simulink model "untitled"  (R2019b)
settings: Solver=VariableStepAuto  StartTime=0.0  StopTime=2  RelTol=1e-3
undefined symbols (not defined in the file): Ion, Lithium, sigbuilder_block
libraries: powerlib x38, simulink x10, electricdrivelib x4, re_lib x2, mpclib x1
settings Model: Creator=ADHI  LastModifiedBy=ADHI
settings SolverCC: AlgebraicLoopSolver=LineSearch

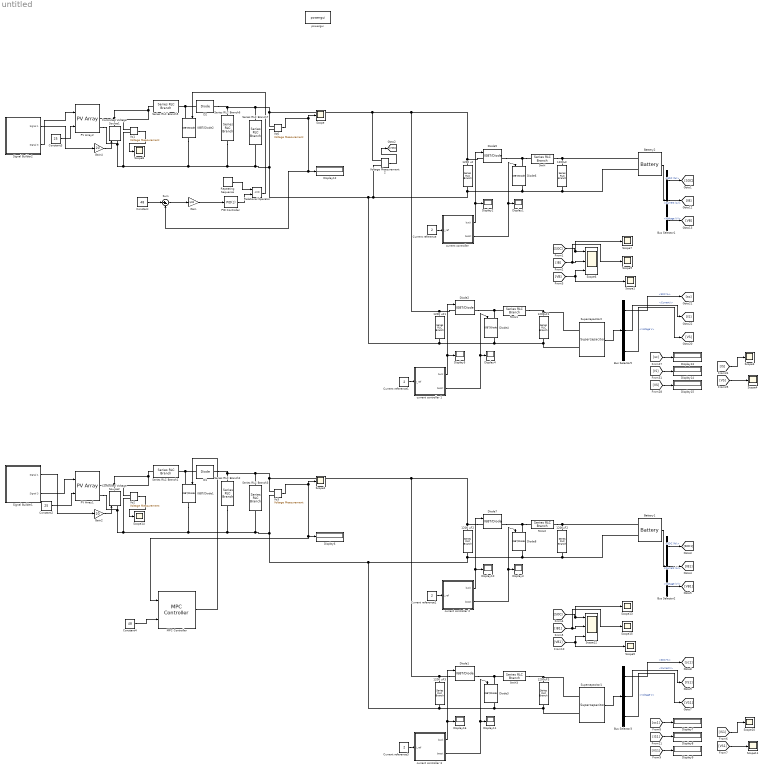
== system untitled ==
  1200 uF : powerlib/Elements/Series RLC Branch  LConnTagsString=__new0  RConnTagsString=__new0  BranchType=RC  Resistance=0.1  Inductance=3e-3  SetiL0=off  InitialCurrent=0  Capacitance=1200e-6  Setx0=off  InitialVoltage=0  Measurements=None
  1200 uF1 : powerlib/Elements/Series RLC Branch  LConnTagsString=__new0  RConnTagsString=__new0  BranchType=RC  Resistance=1  Inductance=3e-3  SetiL0=off  InitialCurrent=0  Capacitance=120e-6  Setx0=off  InitialVoltage=0  Measurements=None
  1200 uF2 : powerlib/Elements/Series RLC Branch  LConnTagsString=__new0  RConnTagsString=__new0  BranchType=RC  Resistance=0.1  Inductance=3e-3  SetiL0=off  InitialCurrent=0  Capacitance=1200e-6  Setx0=off  InitialVoltage=0  Measurements=None
  1200 uF3 : powerlib/Elements/Series RLC Branch  LConnTagsString=__new0  RConnTagsString=__new0  BranchType=RC  Resistance=1  Inductance=3e-3  SetiL0=off  InitialCurrent=0  Capacitance=120e-6  Setx0=off  InitialVoltage=0  Measurements=None
  1200uF : powerlib/Elements/Series RLC Branch  LConnTagsString=__new0  RConnTagsString=__new0  BranchType=C  Resistance=1  Inductance=3e-3  SetiL0=off  InitialCurrent=0  Capacitance=1200e-6  Setx0=off  InitialVoltage=0  Measurements=None
  1200uF1 : powerlib/Elements/Series RLC Branch  LConnTagsString=__new0  RConnTagsString=__new0  BranchType=C  Resistance=1  Inductance=3e-3  SetiL0=off  InitialCurrent=0  Capacitance=120e-6  Setx0=off  InitialVoltage=0  Measurements=None
  1200uF2 : powerlib/Elements/Series RLC Branch  LConnTagsString=__new0  RConnTagsString=__new0  BranchType=C  Resistance=1  Inductance=3e-3  SetiL0=off  InitialCurrent=0  Capacitance=1200e-6  Setx0=off  InitialVoltage=0  Measurements=None
  1200uF3 : powerlib/Elements/Series RLC Branch  LConnTagsString=__new0  RConnTagsString=__new0  BranchType=C  Resistance=1  Inductance=3e-3  SetiL0=off  InitialCurrent=0  Capacitance=120e-6  Setx0=off  InitialVoltage=0  Measurements=None
  9mH : powerlib/Elements/Series RLC Branch  LConnTagsString=__new0  RConnTagsString=__new0  BranchType=L  Resistance=1  Inductance=9e-3  SetiL0=off  InitialCurrent=0  Capacitance=1e-6  Setx0=off  InitialVoltage=0  Measurements=None
  9mH1 : powerlib/Elements/Series RLC Branch  LConnTagsString=__new0  RConnTagsString=__new0  BranchType=L  Resistance=1  Inductance=9e-6  SetiL0=off  InitialCurrent=0  Capacitance=1e-6  Setx0=off  InitialVoltage=0  Measurements=None
  9mH2 : powerlib/Elements/Series RLC Branch  LConnTagsString=__new0  RConnTagsString=__new0  BranchType=L  Resistance=1  Inductance=9e-3  SetiL0=off  InitialCurrent=0  Capacitance=1e-6  Setx0=off  InitialVoltage=0  Measurements=None
  9mH3 : powerlib/Elements/Series RLC Branch  LConnTagsString=__new0  RConnTagsString=__new0  BranchType=L  Resistance=1  Inductance=9e-6  SetiL0=off  InitialCurrent=0  Capacitance=1e-6  Setx0=off  InitialVoltage=0  Measurements=None
  Battery1 : electricdrivelib/Extra Sources/Battery  BatType=Lithium-Ion  ShowTempParam=off  ThermalPreset=no  ShowAgeParam=off  NomV=1.2  NomQ=6.5  SOC=50  Batt_Tr=1e-6  PresetModel=off  MaxQ=7  MinV=50  FullV=1.39  Dis_rate=1.3  R=2  Normal_OP=6.25  expZone=[1.28,1.3]  current=[1.5 3 6]  Units=Time  Tci=20  NomT=20  T2=-30  MaxQ2=4.8  FullV2=7.1  Normal_OP2=5.655  expZone2="[6.58           1]"  Rca=0.6  ti=2000  Dp=0  Neq0=0  Tsim=1e6  Ta1=25  Qeol=5.4*0.9  Reol=0.013333*1.2  Char_age=[2.3478, 3]  Dis_age=[2.3478, 10]  N1=1500  N2=10500  N3=1000  N4=1400  Ta2=45  N5=950
      settings: SourceProductName=Simscape Electrical
  Battery2 : electricdrivelib/Extra Sources/Battery  BatType=Lithium-Ion  ShowTempParam=off  ThermalPreset=no  ShowAgeParam=off  NomV=1.2  NomQ=6.5  SOC=50  Batt_Tr=1e-6  PresetModel=off  MaxQ=7  MinV=50  FullV=1.39  Dis_rate=1.3  R=2  Normal_OP=6.25  expZone=[1.28,1.3]  current=[1.5 3 6]  Units=Time  Tci=20  NomT=20  T2=-30  MaxQ2=4.8  FullV2=7.1  Normal_OP2=5.655  expZone2="[6.58           1]"  Rca=0.6  ti=2000  Dp=0  Neq0=0  Tsim=1e6  Ta1=25  Qeol=5.4*0.9  Reol=0.013333*1.2  Char_age=[2.3478, 3]  Dis_age=[2.3478, 10]  N1=1500  N2=10500  N3=1000  N4=1400  Ta2=45  N5=950
      settings: SourceProductName=Simscape Electrical
  Bus Selector1 : BusSelector  OutputSignals=SOC (%),Current (A),Voltage (V)
  Bus Selector2 : BusSelector  OutputSignals=SOC (%),Current (A),Voltage (V)
  Bus Selector3 : BusSelector  OutputSignals=SOC %,Current I,Voltage V
  Bus Selector5 : BusSelector  OutputSignals=SOC %,Current I,Voltage V
  Constant : Constant  Value=48
  Constant2 : Constant  Value=25
  Constant3 : Constant  Value=25
  Constant4 : Constant  Value=48
  Controlled Voltage Source1 : powerlib/Electrical Sources/Controlled Voltage Source  Initialize=on  Source_Type=DC  Amplitude=5  Phase=0  Frequency=0  Measurements=None
      settings: SourceProductName=Simscape Electrical
  Controlled Voltage Source2 : powerlib/Electrical Sources/Controlled Voltage Source  Initialize=on  Source_Type=DC  Amplitude=5  Phase=0  Frequency=0  Measurements=None
      settings: SourceProductName=Simscape Electrical
  Current reference{,1..3} (4 alike) : Constant  Value=2
  D1 : powerlib/Power Electronics/Diode  Ron=0.001  Lon=0  Vf=0.001  IC=0  UseSnubber=off  Rs=500  Cs=250e-9  Measurements=off
      settings: SourceProductName=Simscape Electrical
  D2 : powerlib/Power Electronics/Diode  Ron=0.001  Lon=0  Vf=0.001  IC=0  UseSnubber=off  Rs=500  Cs=250e-9  Measurements=off
      settings: SourceProductName=Simscape Electrical
  Diode{1..8} (8 alike) : powerlib/Power Electronics/IGBT//Diode  Ron=1e-3  Rs=1e5  Cs=inf  Measurements=on
  Display{1..16} (16 alike) : Display
  Gain : Gain  Gain=1/20
  Gain2 : Gain  Gain=20
  Gain4 : Gain  Gain=20
  IGBT/Diode1 : powerlib/Power Electronics/IGBT//Diode  Ron=1e-3  Rs=1e5  Cs=inf  Measurements=off
      settings: SourceProductName=Simscape Electrical
  IGBT/Diode2 : powerlib/Power Electronics/IGBT//Diode  Ron=1e-3  Rs=1e5  Cs=inf  Measurements=off
      settings: SourceProductName=Simscape Electrical
  MPC Controller : mpclib/MPC Controller  SCDEnableBlockLinearizationSpecification=on  is_multiple=0  enable_value=0  return_u0=off  updateMPCinCallerWorkspace=on  md_inport=off  mv_inport=off  uref_inport=off  return_cost=off  return_mvseq=off  return_qpstatus=off  return_xseq=off  return_state=off  return_ovseq=off  state_inport=off  umin_inport=off  umax_inport=off  ymin_inport=off  ymax_inport=off  cc_inport=off  ywt_inport=off  uwt_inport=off  duwt_inport=off  rhoeps_inport=off  pm_inport=off  MaximumP=10  HorizonChoice=FixedHorizon  n_ts=1  n_p=10  n_mv=1  n_md=1  n_ud=0  n_mo=1  n_uo=0  BlockDataType=double  SampleTimeInherited=off  switch_inport=off
  PID Controller : simulink/Continuous/PID Controller  Controller=PID  Form=Parallel  TimeDomain=Discrete-time  SampleTime=-1  IntegratorMethod=Forward Euler  FilterMethod=Forward Euler  ControllerParametersSource=internal  P=0.7  I=100  D=0  UseFilter=on  N=100  TunerSelectOption=Transfer Function Based (PID Tuner App)  InitialConditionSource=internal  InitialConditionForIntegrator=0  InitialConditionForFilter=0  DifferentiatorICPrevScaledInput=0  ExternalReset=none  TrackingMode=off  Kt=1  LimitOutput=on  UpperSaturationLimit=0.9  LowerSaturationLimit=0.1  LinearizeAsGain=on  AntiWindupMode=none  Kb=1  POutMin=[]  POutMax=[]  IOutMin=[]  IOutMax=[]  DOutMin=[]  DOutMax=[]  NOutMin=[]  NOutMax=[]  SumOutMin=[]  SumOutMax=[]  SaturationOutMin=[]  SaturationOutMax=[]  PParamMin=[]  PParamMax=[]  IParamMin=[]  IParamMax=[]  DParamMin=[]  DParamMax=[]  NParamMin=[]  NParamMax=[]  KbParamMin=[]  KbParamMax=[]  KtParamMin=[]  KtParamMax=[]  KbOutMin=[]  KbOutMax=[]  KtOutMin=[]  KtOutMax=[]  IntegratorOutMin=[]  IntegratorOutMax=[]  FilterOutMin=[]  FilterOutMax=[]  SumI1OutMin=[]  SumI1OutMax=[]  SumI2OutMin=[]  SumI2OutMax=[]  SumI3OutMin=[]  SumI3OutMax=[]  SumI4OutMin=[]  SumI4OutMax=[]  SumDOutMin=[]  SumDOutMax=[]  DifferentiatorOutMin=[]  DifferentiatorOutMax=[]  FilterDiffOutCoefMin=[]  FilterDiffOutCoefMax=[]  ReciprocalOutMin=[]  ReciprocalOutMax=[]  SumDenOutMin=[]  SumDenOutMax=[]  SumNumOutMin=[]  SumNumOutMax=[]  DivideOutMin=[]  DivideOutMax=[]  IntegratorContinuousStateAttributes=''  IntegratorStateMustResolveToSignalObject=off  IntegratorRTWStateStorageClass=Auto  FilterContinuousStateAttributes=''  FilterStateMustResolveToSignalObject=off  FilterRTWStateStorageClass=Auto  ParallelPVariant=InternalParameters  IdealPVariant=Disabled  IVariant=InternalParameters  DVariant=InternalParameters  IntegratorVariant=Discrete  SatVariant=Enabled  AWVariant=Passthrough  PCopyVariant=Disabled  TRVariant=Disabled  FdbkBlocksVariant=Forward  IdealPFdbkVariant=Disabled  SatFdbkVariant=Disabled  DerivativeFilterVariant=ForwardEulerFilter  NVariant=InternalParameters  NCopyVariant=Disabled  FilterICVariant=InternalICsFilter  IntegratorICVariant=InternalICs  ExternalResetVariant=Disabled  TRSumVariant=Passthrough  SumFdbkVariant=Disabled  SumVariant=Sum_PID
  PV Array1 : re_lib/Solar/PV Array  Npar=1  Nser=2  PlotType=array @ 1000 W/m2 & specified temperatures  S_vec="[ 1000  500  100 ]"  Temp_C_vec="[ 45 25  ]"  ModuleName=1Soltech 1STH-340-WH  PlotWhenSelected=off  Pm=339.78  Ncell=80  Voc=51.1  Isc=9.12  Vm=42  Im=8.09  beta_Voc_pc=-0.36  alpha_Isc_pc=0.09  beta_Voc=-0.18396  alpha_Isc=0.008208  IL=9.1647  I0=3.1652e-10  nI=1.0358  Rsh=66.7455  Rs=0.32744  BAL=off  Tc=1e-6  Tfilter=5e-5
      settings: SourceProductName=Simscape Electrical
  PV Array2 : re_lib/Solar/PV Array  Npar=1  Nser=2  PlotType=array @ 1000 W/m2 & specified temperatures  S_vec="[ 1000  500  100 ]"  Temp_C_vec="[ 45 25  ]"  ModuleName=1Soltech 1STH-340-WH  PlotWhenSelected=off  Pm=339.78  Ncell=80  Voc=51.1  Isc=9.12  Vm=42  Im=8.09  beta_Voc_pc=-0.36  alpha_Isc_pc=0.09  beta_Voc=-0.18396  alpha_Isc=0.008208  IL=9.1647  I0=3.1652e-10  nI=1.0358  Rsh=66.7455  Rs=0.32744  BAL=off  Tc=1e-6  Tfilter=5e-5
      settings: SourceProductName=Simscape Electrical
  Relational Operator : RelationalOperator  Operator=<=  OutDataTypeStr=boolean  RndMeth=Simplest
  Repeating Sequence : simulink/Sources/Repeating Sequence  rep_seq_t=[0 0.00004]  rep_seq_y=[0 1]
  Scope{,1..5,7..11,13..15} (14 alike) : Scope
  Scope12 : Scope  NumInputPorts=3
  Scope6 : Scope  NumInputPorts=3
  Series RLC Branch1 : powerlib/Elements/Series RLC Branch  LConnTagsString=__new0  RConnTagsString=__new0  BranchType=L  Resistance=1  Inductance=150e-9  SetiL0=off  InitialCurrent=0  Capacitance=1e-6  Setx0=off  InitialVoltage=0  Measurements=None
      settings: SourceProductName=Simscape Electrical
  Series RLC Branch2 : powerlib/Elements/Series RLC Branch  LConnTagsString=__new0  RConnTagsString=__new0  BranchType=C  Resistance=1  Inductance=1e-3  SetiL0=off  InitialCurrent=0  Capacitance=360e-6  Setx0=off  InitialVoltage=0  Measurements=None
      settings: SourceProductName=Simscape Electrical
  Series RLC Branch3 : powerlib/Elements/Series RLC Branch  LConnTagsString=__new0  RConnTagsString=__new0  BranchType=R  Resistance=10  Inductance=1e-3  SetiL0=off  InitialCurrent=0  Capacitance=220e-6  Setx0=off  InitialVoltage=0  Measurements=None
      settings: SourceProductName=Simscape Electrical
  Series RLC Branch5 : powerlib/Elements/Series RLC Branch  LConnTagsString=__new0  RConnTagsString=__new0  BranchType=L  Resistance=1  Inductance=150e-9  SetiL0=off  InitialCurrent=0  Capacitance=1e-6  Setx0=off  InitialVoltage=0  Measurements=None
      settings: SourceProductName=Simscape Electrical
  Series RLC Branch6 : powerlib/Elements/Series RLC Branch  LConnTagsString=__new0  RConnTagsString=__new0  BranchType=C  Resistance=1  Inductance=1e-3  SetiL0=off  InitialCurrent=0  Capacitance=360e-6  Setx0=off  InitialVoltage=0  Measurements=None
      settings: SourceProductName=Simscape Electrical
  Series RLC Branch7 : powerlib/Elements/Series RLC Branch  LConnTagsString=__new0  RConnTagsString=__new0  BranchType=R  Resistance=10  Inductance=1e-3  SetiL0=off  InitialCurrent=0  Capacitance=220e-6  Setx0=off  InitialVoltage=0  Measurements=None
      settings: SourceProductName=Simscape Electrical
  Signal Builder1 : Subsystem  Tag=STV Subsys  LoadFcn=sigbuilder_block('load');  StartFcn=sigbuilder_block('start');  StopFcn=sigbuilder_block('stop');  ClipboardFcn=sigbuilder_block('clipboard');  mask(Sigbuilder block){tuvar=[0:10]}
      mask help: Simulink:masks:SigbuilderBlock_MD
      mask init:
      | if ~strcmp(get_param(bdroot(gcbh),'SimulationStatus'),'stopped') tuvar = sigbuilder_block('maskInit'); end
      settings: CopyFcn=sigbuilder_block('copy');  DeleteFcn=sigbuilder_block('delete');  ModelCloseFcn=sigbuilder_block('modelClose');  PreSaveFcn=sigbuilder_block('preSave');  PauseFcn=sigbuilder_block('pause');  ContinueFcn=sigbuilder_block('continue');  NameChangeFcn=sigbuilder_block('namechange');  OpenFcn=sigbuilder_block('open',[437.6 153 550.4 359.25 ]);  CloseFcn=sigbuilder_block('close');
      mask Display: plot(0, 0, 100, 100,[2, 2, 32, 32, 2], [68, 8, 8, 68, 68],[32, 2], [38, 38], [32, 19, 2],[53, 60, 44], [32, 17, 17, 2],[16, 16, 31, 31]);txt = getActiveGroup(gcbh);text(2, 100, txt,'verticalAlignment', 'top');
  Signal Builder2 : Subsystem  Tag=STV Subsys  LoadFcn=sigbuilder_block('load');  StartFcn=sigbuilder_block('start');  StopFcn=sigbuilder_block('stop');  ClipboardFcn=sigbuilder_block('clipboard');  mask(Sigbuilder block){tuvar=[0:10]}
      mask help: Simulink:masks:SigbuilderBlock_MD
      mask init:
      | if ~strcmp(get_param(bdroot(gcbh),'SimulationStatus'),'stopped') tuvar = sigbuilder_block('maskInit'); end
      settings: CopyFcn=sigbuilder_block('copy');  DeleteFcn=sigbuilder_block('delete');  ModelCloseFcn=sigbuilder_block('modelClose');  PreSaveFcn=sigbuilder_block('preSave');  PauseFcn=sigbuilder_block('pause');  ContinueFcn=sigbuilder_block('continue');  NameChangeFcn=sigbuilder_block('namechange');  OpenFcn=sigbuilder_block('open',[437.6 153 550.4 359.25 ]);  CloseFcn=sigbuilder_block('close');
      mask Display: plot(0, 0, 100, 100,[2, 2, 32, 32, 2], [68, 8, 8, 68, 68],[32, 2], [38, 38], [32, 19, 2],[53, 60, 44], [32, 17, 17, 2],[16, 16, 31, 31]);txt = getActiveGroup(gcbh);text(2, 100, txt,'verticalAlignment', 'top');
  Sum : Sum  Inputs=|+-
  Supercapacitor1 : electricdrivelib/Extra Sources/Supercapacitor  C=29  Rdc=10  Voltage=48  Ns=1  Np=4  Vinit=48  Temp=25  PresetModel=off  EstParam=off  Nc=1  r=1e-9  epsilon=6.0208e-10  Ich=10  Vstern="[0.161  2.7  7.8]"  Self_dis=on  Ioc=10  Vself="[48  47.8  47.06  44.65]"  demandeplot=off  I="[10  20 100  500]"  Units=sec  Vmax=0  If=0  deltaV=0  alpha=0  sec=0
      settings: SourceProductName=Simscape Power Systems  SourceProductBaseCode=PS
  Supercapacitor2 : electricdrivelib/Extra Sources/Supercapacitor  C=29  Rdc=10  Voltage=48  Ns=1  Np=4  Vinit=48  Temp=25  PresetModel=off  EstParam=off  Nc=1  r=1e-9  epsilon=6.0208e-10  Ich=10  Vstern="[0.161  2.7  7.8]"  Self_dis=on  Ioc=10  Vself="[48  47.8  47.06  44.65]"  demandeplot=off  I="[10  20 100  500]"  Units=sec  Vmax=0  If=0  deltaV=0  alpha=0  sec=0
      settings: SourceProductName=Simscape Power Systems  SourceProductBaseCode=PS
  Vo{1..3,6} (4 alike) : powerlib/Measurements/Voltage Measurement  PhasorSimulation=off  OutputType=Complex  PSBequivalent=0
      settings: SourceProductName=Simscape Electrical
  Voltage Measurement2 : powerlib/Measurements/Voltage Measurement  PhasorSimulation=off  OutputType=Complex  PSBequivalent=0
      settings: SourceProductName=Simscape Electrical
  "current controller " : Subsystem
  current controller 1 : Subsystem
  current controller 2 : Subsystem
  current controller 3 : Subsystem
  powergui : powerlib/powergui  Priority=1  SimulationMode=Discrete  SampleTime=1e-6  frequency=60  Iterations=50  frequencyindice=0  Pbase=100e6  ErrMax=1e-4  UnitsV=kV  UnitsW=MW  buscounter=0  FunctionMessages=off  echomessages=off  EnableUseOfTLC=off  CurrentSourceSwitches=off  DisableSnubberDevices=off  DisableRonSwitches=off  DisableVfSwitches=off  DisplayEquations=off  AutomaticDiscreteSolvers=off  SolverType=Tustin/Backward Euler (TBE)  Interpol=off  ExternalGateDelay=off  methode=off  Ts=100  x0status=blocks  SPID=on  SwTol=0  HookPort=off  NonlinearTolerance=1e-4  nMaxIteration=100  ContinueOnMaxIteration=off  RestoreLinks=warning  ResistiveCurrentMeasurement=off  Frange=[0:2:500]  Ylog=off  Xlog=on  ShowGrid=off  save=off  variable=ZData  structure=0  ZoomFFT=off  StartTime=0.0  cycles=1  DisplayStyle=1  fundamental=60  FreqAxis=off  MaxFrequency=1000  frequencyindicesteady=1  RmsSteady=1  display=off
      settings: SourceProductName=Simscape Electrical
  wires:
  Sum/1 -> Gain/1
  Gain/1 -> PID Controller/1
  Repeating Sequence/1 -> Relational Operator/1
  PID Controller/1 -> Relational Operator/2
  Constant/1 -> Sum/1
  Vo6/1 -> Scope/1, Sum/2, Display12/1
  Vo1/1 -> Scope8/1
  Relational Operator/1 -> IGBT/Diode2/1
  Bus Selector5/1 -> [sc]  "<SOC %>"
  Bus Selector5/3 -> [VS]  "<Voltage V>"
  Battery2/1 -> Bus Selector1/1
  Voltage Measurement2/1 -> [VDC]
  "current controller "/2(boost) -> Display1/1, Diode6/1
  [sc] -> Display13/1
  Current reference/1 -> "current controller "/1(I_ref)
  Bus Selector5/2 -> [IS]  "<Current I>"
  Bus Selector1/3 -> [VB]  "<Voltage (V)>"
  [VB] -> Scope6/3, Scope1/1
  Bus Selector1/2 -> [IB]  "<Current (A)>"
  [SOC] -> Scope6/1, Scope7/1
  Bus Selector1/1 -> [SOC]  "<SOC (%)>"
  Supercapacitor2/1 -> Bus Selector5/1
  current controller 1/1(buck) -> Display5/1, Diode2/1
  current controller 1/2(boost) -> Diode4/1, Display4/1
  [IS] -> Display14/1
  Current reference1/1 -> current controller 1/1(I_ref)
  [IB] -> Scope6/2, Scope9/1
  "current controller "/1(buck) -> Diode5/1, Display2/1
  [VS] -> Display15/1
  [IS] -> Scope3/1
  [VS] -> Scope4/1
  Gain4/1 -> Controlled Voltage Source1/1
  Signal Builder2/1(Signal 1) -> Gain4/1
  Constant3/1 -> PV Array2/2
  Signal Builder2/2(Signal 3) -> PV Array2/1
  Signal Builder1/2(Signal 3) -> PV Array1/1
  Constant2/1 -> PV Array1/2
  Gain2/1 -> Controlled Voltage Source2/1
  [VS1] -> Scope11/1
  [IS1] -> Scope10/1
  [VS1] -> Display9/1
  current controller 2/1(buck) -> Display10/1, Diode7/1
  [IB1] -> Scope15/1, Scope12/2
  Current reference3/1 -> current controller 3/1(I_ref)
  [IS1] -> Display8/1
  current controller 3/2(boost) -> Display11/1, Diode3/1
  current controller 3/1(buck) -> Diode1/1, Display16/1
  Supercapacitor1/1 -> Bus Selector3/1
  Bus Selector2/1 -> [SOC1]  "<SOC (%)>"
  [SOC] -> Scope13/1, Scope12/1
  Bus Selector2/2 -> [IB1]  "<Current (A)>"
  [VB1] -> Scope5/1, Scope12/3
  Bus Selector2/3 -> [VB1]  "<Voltage (V)>"
  Bus Selector3/2 -> [IS1]  "<Current I>"
  Current reference2/1 -> current controller 2/1(I_ref)
  [sc1] -> Display7/1
  current controller 2/2(boost) -> Diode8/1, Display3/1
  Battery1/1 -> Bus Selector2/1
  Bus Selector3/3 -> [VS1]  "<Voltage V>"
  Bus Selector3/1 -> [sc1]  "<SOC %>"
  Vo2/1 -> Scope14/1
  Vo3/1 -> MPC Controller/1, Display6/1, Scope2/1
  Constant4/1 -> MPC Controller/2
  Signal Builder1/1(Signal 1) -> Gain2/1
  MPC Controller/1 -> IGBT/Diode1/1
  connections:
  1200uF1/RConn1 -- Supercapacitor2/LConn2 -- 1200 uF/RConn1 -- Diode6/RConn1 -- Battery2/LConn2 -- 1200uF/RConn1 -- Voltage Measurement2/LConn2 -- Vo6/LConn2 -- IGBT/Diode2/RConn1 -- PV Array2/RConn2 -- Controlled Voltage Source1/LConn1 -- Vo1/LConn2 -- Series RLC Branch6/RConn1 -- Series RLC Branch7/RConn1 -- 1200 uF1/RConn1 -- Diode4/RConn1
  1200 uF1/LConn1 -- 1200 uF/LConn1 -- Diode5/LConn1 -- Voltage Measurement2/LConn1 -- D2/RConn1 -- Series RLC Branch6/LConn1 -- Series RLC Branch7/LConn1 -- Vo6/LConn1 -- Diode2/LConn1
  Series RLC Branch5/RConn1 -- D2/LConn1 -- IGBT/Diode2/LConn1
  Series RLC Branch5/LConn1 -- PV Array2/RConn1 -- Controlled Voltage Source1/RConn1 -- Vo1/LConn1
  9mH1/RConn1 -- Supercapacitor2/LConn1 -- 1200uF1/LConn1
  9mH/LConn1 -- Diode6/LConn1 -- Diode5/RConn1
  1200uF/LConn1 -- Battery2/LConn1 -- 9mH/RConn1
  Diode4/LConn1 -- 9mH1/LConn1 -- Diode2/RConn1
  1200uF3/RConn1 -- Diode3/RConn1 -- 1200 uF3/RConn1 -- 1200uF2/RConn1 -- Battery1/LConn2 -- Diode8/RConn1 -- 1200 uF2/RConn1 -- Series RLC Branch3/RConn1 -- Series RLC Branch2/RConn1 -- Vo2/LConn2 -- Controlled Voltage Source2/LConn1 -- PV Array1/RConn2 -- IGBT/Diode1/RConn1 -- Vo3/LConn2 -- Supercapacitor1/LConn2
  1200 uF3/LConn1 -- Diode1/LConn1 -- Vo3/LConn1 -- Series RLC Branch3/LConn1 -- Series RLC Branch2/LConn1 -- D1/RConn1 -- Diode7/LConn1 -- 1200 uF2/LConn1
  Series RLC Branch1/RConn1 -- IGBT/Diode1/LConn1 -- D1/LConn1
  Series RLC Branch1/LConn1 -- Vo2/LConn1 -- Controlled Voltage Source2/RConn1 -- PV Array1/RConn1
  9mH3/RConn1 -- 1200uF3/LConn1 -- Supercapacitor1/LConn1
  9mH2/LConn1 -- Diode7/RConn1 -- Diode8/LConn1
  Battery1/LConn1 -- 9mH2/RConn1 -- 1200uF2/LConn1
  Diode3/LConn1 -- Diode1/RConn1 -- 9mH3/LConn1

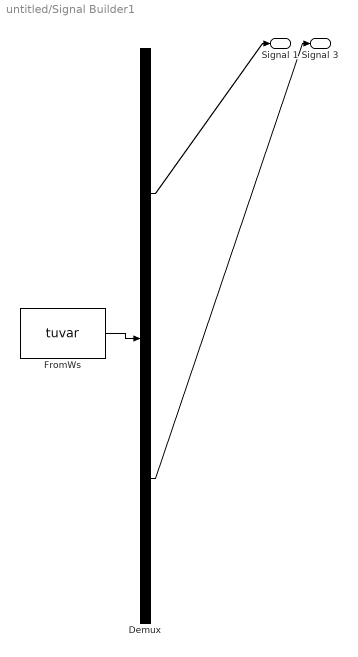
== system untitled/Signal Builder1 ==
  Demux : Demux  Tag=STV Demux  Outputs=2
  FromWs : FromWorkspace  Tag=STV FromWs  VariableName=tuvar  SampleTime=0
      SigBuilderData=|
      | common.afterFinalStr = 'Extrapolate'
      | common.sampleTime = 0
      | dataSet.timeRange = [0 4]
      | dataSet.name = 'Group 1'
      | sbobj.Groups.Name = 'Group 1'
      | sbobj.Groups.Signals(1).Name = 'Signal 1'
      | sbobj.Groups.Signals(1).XData = [0 0.5 0.5 1 1 4]
      | sbobj.Groups.Signals(1).YData = [2.3 2.3 2.316 2.316 2.3 2.3]
      | sbobj.Groups.Signals(2).Name = 'Signal 3'
      | sbobj.Groups.Signals(2).XData = [0 0.5 0.5 1 1 4]
      | sbobj.Groups.Signals(2).YData = [300 300 450 450 300 300]
      | sbobj.Groups.TimeRange = [0 4]
  Signal 1 : Outport  Tag=STV Outport
  Signal 3 : Outport  Tag=STV Outport  Port=2
  wires:
  Demux/2 -> Signal 3/1
  Demux/1 -> Signal 1/1
  FromWs/1 -> Demux/1

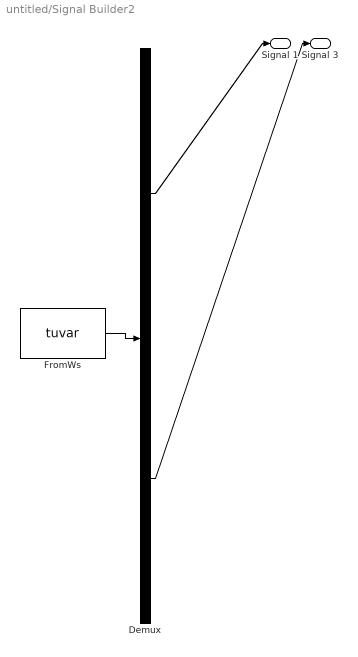
== system untitled/Signal Builder2 ==
  Demux : Demux  Tag=STV Demux  Outputs=2
  FromWs : FromWorkspace  Tag=STV FromWs  VariableName=tuvar  SampleTime=0
      SigBuilderData=|
      | common.afterFinalStr = 'Extrapolate'
      | common.sampleTime = 0
      | dataSet.timeRange = [0 4]
      | dataSet.name = 'Group 1'
      | sbobj.Groups.Name = 'Group 1'
      | sbobj.Groups.Signals(1).Name = 'Signal 1'
      | sbobj.Groups.Signals(1).XData = [0 0.5 0.5 1 1 4]
      | sbobj.Groups.Signals(1).YData = [0.49 0.49 0.84 0.84 0.5 0.5]
      | sbobj.Groups.Signals(2).Name = 'Signal 3'
      | sbobj.Groups.Signals(2).XData = [0 0.5 0.5 1 1 4]
      | sbobj.Groups.Signals(2).YData = [300 300 450 450 300 300]
      | sbobj.Groups.TimeRange = [0 4]
  Signal 1 : Outport  Tag=STV Outport
  Signal 3 : Outport  Tag=STV Outport  Port=2
  wires:
  FromWs/1 -> Demux/1
  Demux/1 -> Signal 1/1
  Demux/2 -> Signal 3/1

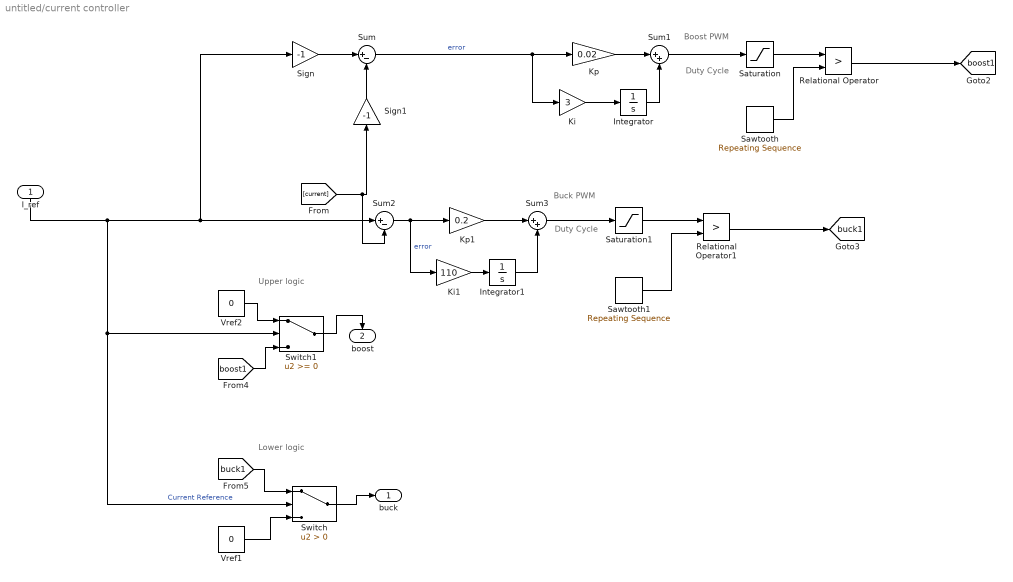
== system untitled/current controller  ==
  note: Buck PWM
  note: Duty Cycle
  note: Upper logic
  note: Lower logic
  note: Boost PWM
  note: Duty Cycle
  I_ref : Inport
  Integrator : Integrator  LimitOutput=on  UpperSaturationLimit=0.9  LowerSaturationLimit=0
  Integrator1 : Integrator  LimitOutput=on  UpperSaturationLimit=0.9  LowerSaturationLimit=0
  Ki : Gain  Gain=3
  Ki1 : Gain  Gain=110
  Kp : Gain  Gain=0.02
  Kp1 : Gain  Gain=0.2
  Relational Operator : RelationalOperator  Operator=>  OutDataTypeStr=boolean  RndMeth=Nearest
  Relational Operator1 : RelationalOperator  Operator=>  OutDataTypeStr=boolean  RndMeth=Nearest
  Saturation : Saturate  UpperLimit=0.9  LowerLimit=0
  Saturation1 : Saturate  UpperLimit=0.8  LowerLimit=0
  Sawtooth : simulink/Sources/Repeating Sequence  rep_seq_t=[0 1/5000]  rep_seq_y=[0 1]
  Sawtooth1 : simulink/Sources/Repeating Sequence  rep_seq_t=[0 1/5000]  rep_seq_y=[0 1]
  Sign : Gain  Gain=-1
  Sign1 : Gain  Gain=-1
  Sum : Sum  Inputs=|+-
  Sum1 : Sum  Inputs=|++
  Sum2 : Sum  Inputs=|+-
  Sum3 : Sum  Inputs=|++
  Switch : Switch  Criteria=u2 > Threshold
  Switch1 : Switch
  Vref1 : Constant  Value=0
  Vref2 : Constant  Value=0
  buck : Outport
  boost : Outport  Port=2
  tag scope: boost1=global, buck1=global
  wires:
  Integrator/1 -> Sum1/2
  Kp/1 -> Sum1/1
  Sum/1 -> Kp/1, Ki/1  "error"
  Relational Operator/1 -> [boost1]
  Sign/1 -> Sum/1
  Sum1/1 -> Saturation/1
  Ki/1 -> Integrator/1
  Sum3/1 -> Saturation1/1
  Integrator1/1 -> Sum3/2
  Sawtooth/1 -> Relational Operator/2
  Sawtooth1/1 -> Relational Operator1/2
  [current] -> Sign1/1, Sum2/2
  Kp1/1 -> Sum3/1
  Relational Operator1/1 -> [buck1]
  Sum2/1 -> Ki1/1, Kp1/1  "error"
  Saturation/1 -> Relational Operator/1
  Saturation1/1 -> Relational Operator1/1
  Ki1/1 -> Integrator1/1
  Switch1/1 -> boost/1
  Vref1/1 -> Switch/3
  Vref2/1 -> Switch1/1
  [boost1] -> Switch1/3
  Switch/1 -> buck/1
  [buck1] -> Switch/1
  I_ref/1 -> Sign/1, Sum2/1, Switch/2, Switch1/2  "Current Reference"
  Sign1/1 -> Sum/2

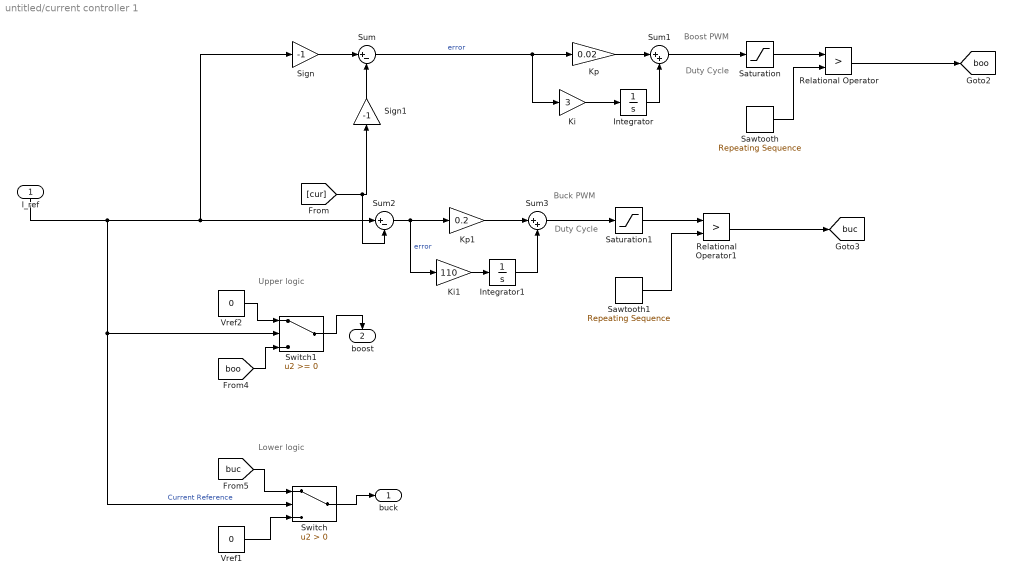
== system untitled/current controller 1 ==
  note: Duty Cycle
  note: Boost PWM
  note: Lower logic
  note: Upper logic
  note: Duty Cycle
  note: Buck PWM
  I_ref : Inport
  Integrator : Integrator  LimitOutput=on  UpperSaturationLimit=0.9  LowerSaturationLimit=0
  Integrator1 : Integrator  LimitOutput=on  UpperSaturationLimit=0.9  LowerSaturationLimit=0
  Ki : Gain  Gain=3
  Ki1 : Gain  Gain=110
  Kp : Gain  Gain=0.02
  Kp1 : Gain  Gain=0.2
  Relational Operator : RelationalOperator  Operator=>  OutDataTypeStr=boolean  RndMeth=Nearest
  Relational Operator1 : RelationalOperator  Operator=>  OutDataTypeStr=boolean  RndMeth=Nearest
  Saturation : Saturate  UpperLimit=0.9  LowerLimit=0
  Saturation1 : Saturate  UpperLimit=0.8  LowerLimit=0
  Sawtooth : simulink/Sources/Repeating Sequence  rep_seq_t=[0 1/5000]  rep_seq_y=[0 1]
  Sawtooth1 : simulink/Sources/Repeating Sequence  rep_seq_t=[0 1/5000]  rep_seq_y=[0 1]
  Sign : Gain  Gain=-1
  Sign1 : Gain  Gain=-1
  Sum : Sum  Inputs=|+-
  Sum1 : Sum  Inputs=|++
  Sum2 : Sum  Inputs=|+-
  Sum3 : Sum  Inputs=|++
  Switch : Switch  Criteria=u2 > Threshold
  Switch1 : Switch
  Vref1 : Constant  Value=0
  Vref2 : Constant  Value=0
  buck : Outport
  boost : Outport  Port=2
  tag scope: boo=global, buc=global
  wires:
  Sign1/1 -> Sum/2
  I_ref/1 -> Switch1/2, Switch/2, Sum2/1, Sign/1  "Current Reference"
  [buc] -> Switch/1
  Switch/1 -> buck/1
  [boo] -> Switch1/3
  Vref2/1 -> Switch1/1
  Vref1/1 -> Switch/3
  Switch1/1 -> boost/1
  Ki1/1 -> Integrator1/1
  Saturation1/1 -> Relational Operator1/1
  Saturation/1 -> Relational Operator/1
  Sum2/1 -> Kp1/1, Ki1/1  "error"
  Relational Operator1/1 -> [buc]
  Kp1/1 -> Sum3/1
  [cur] -> Sum2/2, Sign1/1
  Sawtooth1/1 -> Relational Operator1/2
  Sawtooth/1 -> Relational Operator/2
  Integrator1/1 -> Sum3/2
  Sum3/1 -> Saturation1/1
  Ki/1 -> Integrator/1
  Sum1/1 -> Saturation/1
  Sign/1 -> Sum/1
  Relational Operator/1 -> [boo]
  Sum/1 -> Ki/1, Kp/1  "error"
  Kp/1 -> Sum1/1
  Integrator/1 -> Sum1/2

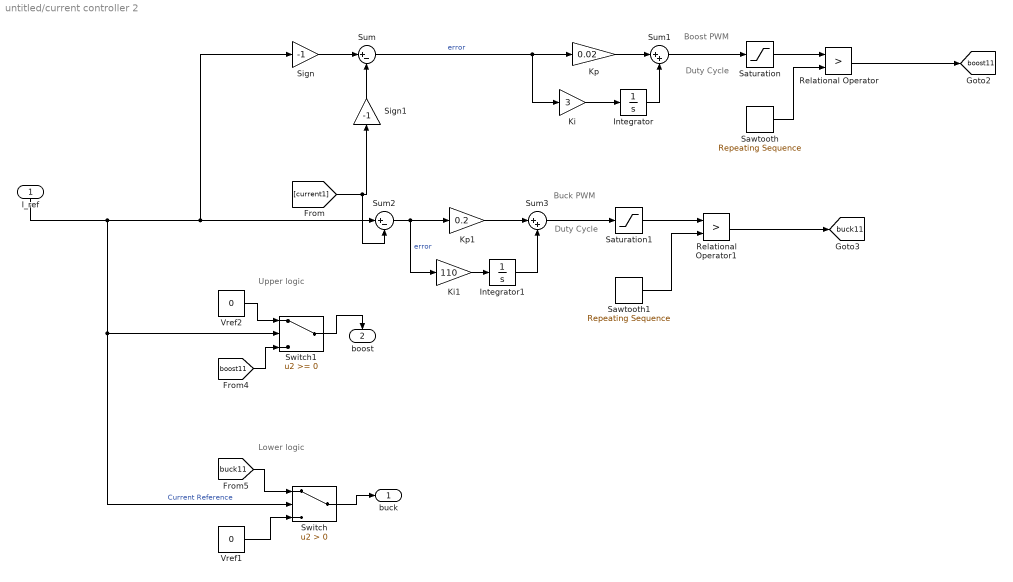
== system untitled/current controller 2 ==
  note: Duty Cycle
  note: Boost PWM
  note: Lower logic
  note: Upper logic
  note: Duty Cycle
  note: Buck PWM
  I_ref : Inport
  Integrator : Integrator  LimitOutput=on  UpperSaturationLimit=0.9  LowerSaturationLimit=0
  Integrator1 : Integrator  LimitOutput=on  UpperSaturationLimit=0.9  LowerSaturationLimit=0
  Ki : Gain  Gain=3
  Ki1 : Gain  Gain=110
  Kp : Gain  Gain=0.02
  Kp1 : Gain  Gain=0.2
  Relational Operator : RelationalOperator  Operator=>  OutDataTypeStr=boolean  RndMeth=Nearest
  Relational Operator1 : RelationalOperator  Operator=>  OutDataTypeStr=boolean  RndMeth=Nearest
  Saturation : Saturate  UpperLimit=0.9  LowerLimit=0
  Saturation1 : Saturate  UpperLimit=0.8  LowerLimit=0
  Sawtooth : simulink/Sources/Repeating Sequence  rep_seq_t=[0 1/5000]  rep_seq_y=[0 1]
  Sawtooth1 : simulink/Sources/Repeating Sequence  rep_seq_t=[0 1/5000]  rep_seq_y=[0 1]
  Sign : Gain  Gain=-1
  Sign1 : Gain  Gain=-1
  Sum : Sum  Inputs=|+-
  Sum1 : Sum  Inputs=|++
  Sum2 : Sum  Inputs=|+-
  Sum3 : Sum  Inputs=|++
  Switch : Switch  Criteria=u2 > Threshold
  Switch1 : Switch
  Vref1 : Constant  Value=0
  Vref2 : Constant  Value=0
  buck : Outport
  boost : Outport  Port=2
  tag scope: boost11=global, buck11=global
  wires:
  Sign1/1 -> Sum/2
  I_ref/1 -> Switch1/2, Switch/2, Sum2/1, Sign/1  "Current Reference"
  [buck11] -> Switch/1
  Switch/1 -> buck/1
  [boost11] -> Switch1/3
  Vref2/1 -> Switch1/1
  Vref1/1 -> Switch/3
  Switch1/1 -> boost/1
  Ki1/1 -> Integrator1/1
  Saturation1/1 -> Relational Operator1/1
  Saturation/1 -> Relational Operator/1
  Sum2/1 -> Kp1/1, Ki1/1  "error"
  Relational Operator1/1 -> [buck11]
  Kp1/1 -> Sum3/1
  [current1] -> Sum2/2, Sign1/1
  Sawtooth1/1 -> Relational Operator1/2
  Sawtooth/1 -> Relational Operator/2
  Integrator1/1 -> Sum3/2
  Sum3/1 -> Saturation1/1
  Ki/1 -> Integrator/1
  Sum1/1 -> Saturation/1
  Sign/1 -> Sum/1
  Relational Operator/1 -> [boost11]
  Sum/1 -> Ki/1, Kp/1  "error"
  Kp/1 -> Sum1/1
  Integrator/1 -> Sum1/2

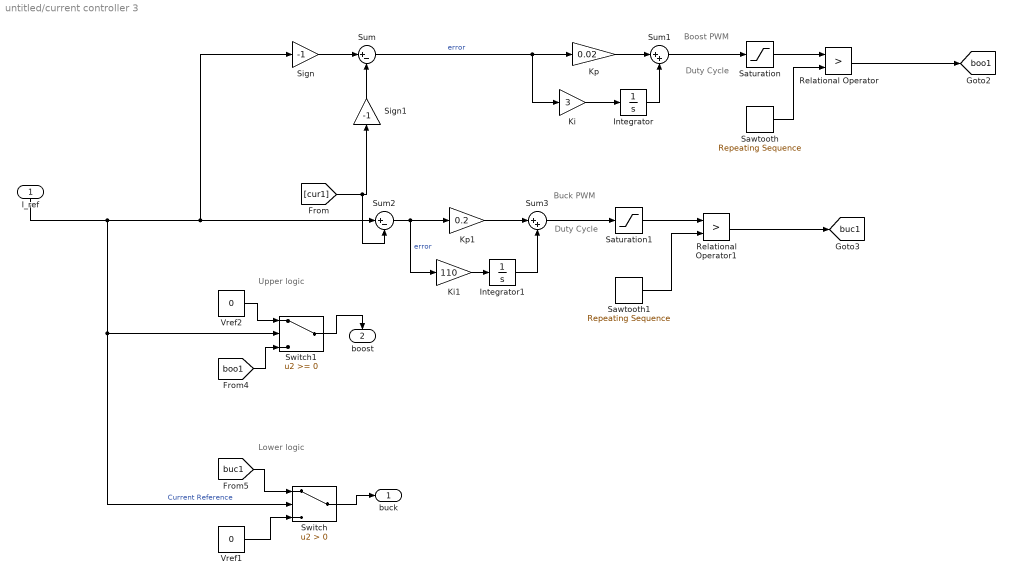
== system untitled/current controller 3 ==
  note: Buck PWM
  note: Duty Cycle
  note: Upper logic
  note: Lower logic
  note: Boost PWM
  note: Duty Cycle
  I_ref : Inport
  Integrator : Integrator  LimitOutput=on  UpperSaturationLimit=0.9  LowerSaturationLimit=0
  Integrator1 : Integrator  LimitOutput=on  UpperSaturationLimit=0.9  LowerSaturationLimit=0
  Ki : Gain  Gain=3
  Ki1 : Gain  Gain=110
  Kp : Gain  Gain=0.02
  Kp1 : Gain  Gain=0.2
  Relational Operator : RelationalOperator  Operator=>  OutDataTypeStr=boolean  RndMeth=Nearest
  Relational Operator1 : RelationalOperator  Operator=>  OutDataTypeStr=boolean  RndMeth=Nearest
  Saturation : Saturate  UpperLimit=0.9  LowerLimit=0
  Saturation1 : Saturate  UpperLimit=0.8  LowerLimit=0
  Sawtooth : simulink/Sources/Repeating Sequence  rep_seq_t=[0 1/5000]  rep_seq_y=[0 1]
  Sawtooth1 : simulink/Sources/Repeating Sequence  rep_seq_t=[0 1/5000]  rep_seq_y=[0 1]
  Sign : Gain  Gain=-1
  Sign1 : Gain  Gain=-1
  Sum : Sum  Inputs=|+-
  Sum1 : Sum  Inputs=|++
  Sum2 : Sum  Inputs=|+-
  Sum3 : Sum  Inputs=|++
  Switch : Switch  Criteria=u2 > Threshold
  Switch1 : Switch
  Vref1 : Constant  Value=0
  Vref2 : Constant  Value=0
  buck : Outport
  boost : Outport  Port=2
  tag scope: boo1=global, buc1=global
  wires:
  Integrator/1 -> Sum1/2
  Kp/1 -> Sum1/1
  Sum/1 -> Kp/1, Ki/1  "error"
  Relational Operator/1 -> [boo1]
  Sign/1 -> Sum/1
  Sum1/1 -> Saturation/1
  Ki/1 -> Integrator/1
  Sum3/1 -> Saturation1/1
  Integrator1/1 -> Sum3/2
  Sawtooth/1 -> Relational Operator/2
  Sawtooth1/1 -> Relational Operator1/2
  [cur1] -> Sign1/1, Sum2/2
  Kp1/1 -> Sum3/1
  Relational Operator1/1 -> [buc1]
  Sum2/1 -> Ki1/1, Kp1/1  "error"
  Saturation/1 -> Relational Operator/1
  Saturation1/1 -> Relational Operator1/1
  Ki1/1 -> Integrator1/1
  Switch1/1 -> boost/1
  Vref1/1 -> Switch/3
  Vref2/1 -> Switch1/1
  [boo1] -> Switch1/3
  Switch/1 -> buck/1
  [buc1] -> Switch/1
  I_ref/1 -> Sign/1, Sum2/1, Switch/2, Switch1/2  "Current Reference"
  Sign1/1 -> Sum/2
